simulink model "s3"  (Simulink 2.00)
settings: Solver=ode15s  StartTime=0.0  StopTime=tstop  MaxStep=1e-3  RelTol=1e-6  AbsTol=1e-6
values from neighbouring files (symbols this model uses):
  Domega = 0    [P20HP.M]
  H = J*wbm*wbm/(2*Sb)    (= 3.33396824273)    [P20HP.M]
  lambdadre = lambdadr.*(invspeed.*mask + notmask)    [M3.M]
  P = 4    [P20HP.M]
  Psidso = 0    [M1C.M]    (also in M1O.M; M3.M)
  Psipdro = 0    [M1C.M]    (also in M1O.M; M3.M)
  Psipqro = 0    [M1C.M]    (also in M1O.M; M3.M)
  Psiqso = 0    [M1C.M]    (also in M1O.M; M3.M)
  rpr = 0.0764    [P20HP.M]
  rs = 0.1062    [P20HP.M]
  speed = wbm*speed    [M3.M]
  speed_wref = [0 0.5 0.5 -0.5 -0.5 0]    [M1C.M]    (also in M1O.M = [0 1 1]; M3.M = [0 wbm/2 wbm/2 -wbm/2 -wbm/2 0])
  Tfactor = (3*P)/(4*wb)    (= 0.00795774715459)    [P20HP.M]
  time_tmech = [0 4]    [M1C.M]    (also in M1O.M = [0 0.75 0.75 1.0 1.0 1.25 1.25 1.5 1.5 2]; M3.M = [0 tstop])
  time_wref = [0 0.25 0.5 1.0 1.25 1.5]    [M1C.M]    (also in M1O.M = [0 0.5 4]; M3.M)
  tmech_tmech = [0 0]    [M1C.M]    (also in M1O.M = [0 0 -Trated -Trated -Trated/2 -Trated/2 -Trated -Trated 0 0; M3.M)
  wb = 2*pi*frated    (= 376.991118431)    [P20HP.M]
  wrbywbo = 0    [M1C.M]    (also in M1O.M; M3.M)
  xls = (we/wb)*xls    [M1C.M]    (also in M1O.M; M3.M; P20HP.M = 0.2145)
  xm = (we/wb)*xm    [M1C.M]    (also in M1O.M; M3.M; P20HP.M = 5.8339)
  xM = 1/(1/xm + 1/xls + 1/xplr)    [M1C.M]    (also in M1O.M; M3.M; P20HP.M = 0.105313916498)
  xplr = (we/wb)*xplr    [M1C.M]    (also in M1O.M; M3.M; P20HP.M = 0.2145)
  xr = xplr + xm    [M1C.M]    (also in M1O.M; M3.M)
  Zb = Vrated*Vrated/Sb    (= 3.24396782842)    [P20HP.M]
settings Model: SaveTime=off  SaveOutput=off  ConsistencyChecking=off

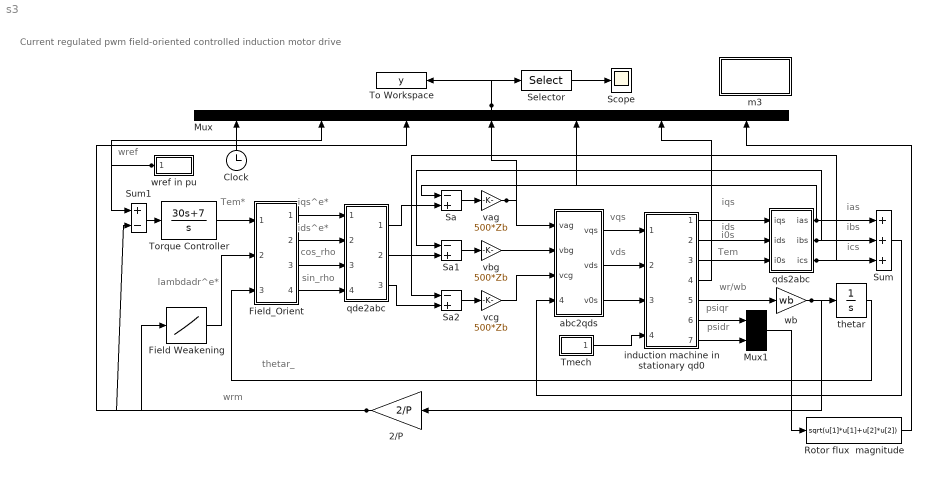
== system s3 ==
  note: Current regulated pwm
      | field-oriented controlled
      | induction motor drive
  note: Tem*
  note: cos_rho
  note: iqs^e*
  note: wref
  note: wrm
  note: thetar_
  note: ids^e*
  note: ics
  note: ibs
  note: ias
  note: vqs
  note: vds
  note: iqs
  note: ids
  note: Tem
  note: wr/wb
  note: i0s
  note: psiqr
  note: psidr
  note: lambdadr^e*
  note: sin_rho
  2/P : Gain  Orientation=left  Gain=2/P
  Clock : Clock
      settings: Orientation=up  DeleteFcn=simclock BlockIsBeingDestroyed  PostSaveFcn=simclock Save
  Field Weakening : Lookup  InputValues=speed  OutputValues=lambdadre
  Field_Orient : Subsystem
  m3 : Subsystem
      settings: OpenFcn=m3
      mask Type: Masked block of m3.m
      mask Help: Uses m3.m to initialize and plot
      mask Display: disp('Initialize\nand plot')
  Mux : Mux  Orientation=up  Inputs=7
  Mux1 : Mux  Inputs=2
  Rotor flux  magnitude : Fcn  Expr=sqrt(u[1]*u[1]+u[2]*u[2])
  Sa : Sum  Inputs=-+
  Sa1 : Sum  Inputs=-+
  Sa2 : Sum  Inputs=-+
  Scope : Scope
      settings: TickLabels=on  TimeRange=2  YMin=-200  YMax=200  SaveToWorkspace=off  SaveName=ScopeData  LimitMaxRows=off
  Selector : Selector  Elements=[3 4 5 6 7]  InputPortWidth=7
  Sum : Sum  Inputs=+++
  Sum1 : Sum  Inputs=+-
  Tmech : Subsystem  mask(Repeating table){rep_seq_t=time_tmech, rep_seq_y=tmech_tmech}
      mask prompts: rep_seq_t "Time values:"; rep_seq_y "Output values:"
      mask help: Repeating table.
      mask init:
      | period = max(rep_seq_t);
      mask Help: Repeats cycle given in table. Time values should be monotonically increasing.
      mask Display: plot([rep_seq_t,rep_seq_t+period,rep_seq_t+2*period,rep_seq_t(1)+3*period],[rep_seq_y,rep_seq_y,rep_seq_y,rep_seq_y(1)])
  To Workspace : ToWorkspace  VariableName=y  SampleTime=0
      settings: Buffer=40000
  Torque Controller : TransferFcn  Numerator=[30 7]  Denominator=[1 0]
  abc2qds : Subsystem
  induction machine in stationary qd0 : Subsystem
  qde2abc : Subsystem
  qds2abc : Subsystem
  thetar : Integrator  ExternalReset=none  InitialConditionSource=internal  InitialCondition=0  LimitOutput=off  UpperSaturationLimit=inf  LowerSaturationLimit=-inf  ShowSaturationPort=off  ShowStatePort=off  AbsoluteTolerance=auto
  vag : Gain  Gain=500*Zb
  vbg : Gain  Gain=500*Zb
  vcg : Gain  Gain=500*Zb
  wb : Gain  Gain=wb
  wref in pu : Subsystem  Orientation=left  mask(Repeating table){rep_seq_t=time_wref, rep_seq_y=speed_wref}
      mask prompts: rep_seq_t "Time values:"; rep_seq_y "Output values:"
      mask help: Repeating table.
      mask init:
      | period = max(rep_seq_t);
      mask Help: Repeats cycle given in table. Time values should be monotonically increasing.
      mask Display: plot([rep_seq_t,rep_seq_t+period,rep_seq_t+2*period,rep_seq_t(1)+3*period],[rep_seq_y,rep_seq_y,rep_seq_y,rep_seq_y(1)])
  wires:
  wref in pu/1(out_1) -> Mux/2, Sum1/1
  Tmech/1(out_1) -> induction machine in stationary qd0/4(in_Tmech)
  Mux/1 -> Selector/1, To Workspace/1
  Selector/1 -> Scope/1
  Sum1/1 -> Torque Controller/1
  Torque Controller/1 -> Field_Orient/1(Tem*)
  vag/1 -> Mux/4, abc2qds/1(vag)
  vcg/1 -> abc2qds/3(vcg)
  vbg/1 -> abc2qds/2(vbg)
  Field Weakening/1 -> Field_Orient/2(lambdadre)
  Rotor flux  magnitude/1 -> Mux/7
  induction machine in stationary qd0/4(out_Tem) -> Mux/6
  qde2abc/2(ibs*) -> Sa1/2
  Mux1/1 -> Rotor flux  magnitude/1
  induction machine in stationary qd0/7(out_psidr) -> Mux1/2
  induction machine in stationary qd0/6(out_psiqr) -> Mux1/1
  Sa2/1 -> vcg/1
  Sa/1 -> vag/1
  Sa1/1 -> vbg/1
  2/P/1 -> Mux/3, Sum1/2, Field Weakening/1
  wb/1 -> 2/P/1, thetar/1
  thetar/1 -> Field_Orient/3(thetar)
  qds2abc/3(ics) -> Sa2/1, Sum/3
  qds2abc/2(ibs) -> Sa1/1, Sum/2
  qds2abc/1(ias) -> Mux/5, Sa/1, Sum/1
  qde2abc/3(ics*) -> Sa2/2
  qde2abc/1(ias*) -> Sa/2
  Field_Orient/4(sin_rho) -> qde2abc/4(sin_rho)
  Field_Orient/3(cos_rho) -> qde2abc/3(cos_rho)
  Field_Orient/2(ids^e*) -> qde2abc/2(ids^e*)
  Field_Orient/1(iqs^e*) -> qde2abc/1(iqs^e*)
  induction machine in stationary qd0/5(out_wr/wb) -> wb/1
  induction machine in stationary qd0/3(out_i0s) -> qds2abc/3(i0s)
  induction machine in stationary qd0/2(out_ids) -> qds2abc/2(ids)
  induction machine in stationary qd0/1(out_iqs) -> qds2abc/1(iqs)
  abc2qds/2(vds) -> induction machine in stationary qd0/2(in_vds)
  Sum/1 -> abc2qds/4(ias+ibs+ics)
  Clock/1 -> Mux/1
  abc2qds/1(vqs) -> induction machine in stationary qd0/1(in_vqs)
  abc2qds/3(v0s) -> induction machine in stationary qd0/3(in_v0s)

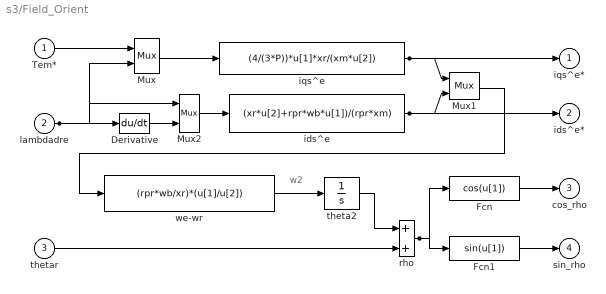
== system s3/Field_Orient ==
  note: w2
  Tem* : Inport  Port=1  PortWidth=-1  SampleTime=-1
  lambdadre : Inport  Port=2  PortWidth=-1  SampleTime=-1
  thetar : Inport  Port=3  PortWidth=-1  SampleTime=-1
  Derivative : Derivative
  Fcn : Fcn  Expr=cos(u[1])
  Fcn1 : Fcn  Expr=sin(u[1])
  Mux : Mux  Inputs=2
  Mux1 : Mux  Inputs=2
  Mux2 : Mux  Inputs=2
  ids^e : Fcn  Expr=(xr*u[2]+rpr*wb*u[1])/(rpr*xm)
  iqs^e : Fcn  Expr=(4/(3*P))*u[1]*xr/(xm*u[2])
  rho : Sum  Inputs=++
  theta2 : Integrator  ExternalReset=none  InitialConditionSource=internal  InitialCondition=0  LimitOutput=off  UpperSaturationLimit=inf  LowerSaturationLimit=-inf  ShowSaturationPort=off  ShowStatePort=off  AbsoluteTolerance=auto
  we-wr : Fcn  Expr=(rpr*wb/xr)*(u[1]/u[2])
  iqs^e* : Outport  Port=1  InitialOutput=0
  ids^e* : Outport  Port=2  InitialOutput=0
  cos_rho : Outport  Port=3  InitialOutput=0
  sin_rho : Outport  Port=4  InitialOutput=0
  wires:
  ids^e/1 -> Mux1/2, ids^e*/1
  Mux2/1 -> ids^e/1
  lambdadre/1 -> Mux2/1, Mux/2, Derivative/1
  Fcn1/1 -> sin_rho/1
  thetar/1 -> rho/2
  Fcn/1 -> cos_rho/1
  iqs^e/1 -> iqs^e*/1, Mux1/1
  Tem*/1 -> Mux/1
  Mux/1 -> iqs^e/1
  Mux1/1 -> we-wr/1
  we-wr/1 -> theta2/1
  theta2/1 -> rho/1
  rho/1 -> Fcn/1, Fcn1/1
  Derivative/1 -> Mux2/2

== system s3/m3 ==
  note: Masked block of m3.m to initialize s3.m
      | and plot results of the simulation

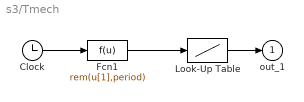
== system s3/Tmech ==
  Clock : Clock
      settings: DeleteFcn=simclock BlockIsBeingDestroyed  PostSaveFcn=simclock Save
  Fcn1 : Fcn  Expr=rem(u[1],period)
  Look-Up Table : Lookup  InputValues=rep_seq_t  OutputValues=rep_seq_y
  out_1 : Outport  Port=1  InitialOutput=0
  wires:
  Look-Up Table/1 -> out_1/1
  Clock/1 -> Fcn1/1
  Fcn1/1 -> Look-Up Table/1

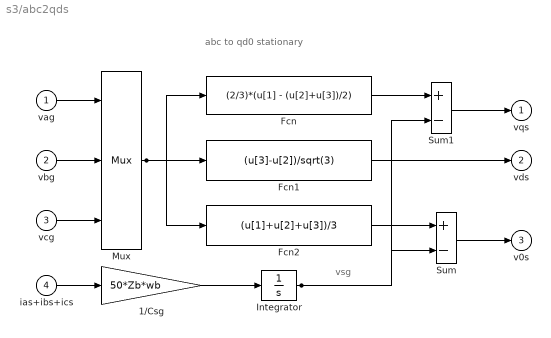
== system s3/abc2qds ==
  note: vsg
  note: abc to qd0 stationary
  vag : Inport  Port=1  PortWidth=-1  SampleTime=-1
  vbg : Inport  Port=2  PortWidth=-1  SampleTime=-1
  vcg : Inport  Port=3  PortWidth=-1  SampleTime=-1
  ias+ibs+ics : Inport  Port=4  PortWidth=-1  SampleTime=-1
  1/Csg : Gain  Gain=50*Zb*wb
  Fcn : Fcn  Expr=(2/3)*(u[1] - (u[2]+u[3])/2)
  Fcn1 : Fcn  Expr=(u[3]-u[2])/sqrt(3)
  Fcn2 : Fcn  Expr=(u[1]+u[2]+u[3])/3
  Integrator : Integrator  ExternalReset=none  InitialConditionSource=internal  InitialCondition=0  LimitOutput=off  UpperSaturationLimit=inf  LowerSaturationLimit=-inf  ShowSaturationPort=off  ShowStatePort=off  AbsoluteTolerance=auto
  Mux : Mux  Inputs=3
  Sum : Sum  Inputs=+-
  Sum1 : Sum  Inputs=+-
  vqs : Outport  Port=1  InitialOutput=0
  vds : Outport  Port=2  InitialOutput=0
  v0s : Outport  Port=3  InitialOutput=0
  wires:
  Integrator/1 -> Sum1/2, Sum/2
  Sum1/1 -> vqs/1
  Fcn/1 -> Sum1/1
  1/Csg/1 -> Integrator/1
  Fcn2/1 -> Sum/1
  Sum/1 -> v0s/1
  Fcn1/1 -> vds/1
  Mux/1 -> Fcn2/1, Fcn/1, Fcn1/1
  vcg/1 -> Mux/3
  vbg/1 -> Mux/2
  vag/1 -> Mux/1
  ias+ibs+ics/1 -> 1/Csg/1

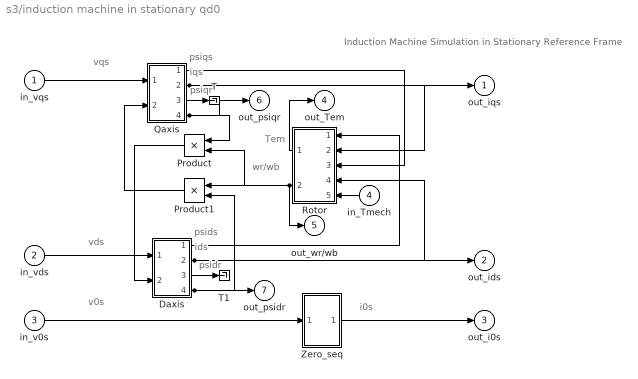
== system s3/induction machine in stationary qd0 ==
  note: Induction Machine Simulation
      |   in Stationary Reference Frame
  note: psiqs
  note: iqs
  note: psiqr
  note: psids
  note: psidr
  note: ids
  note: vqs
  note: vds
  note: wr/wb
  note: Tem
  note: i0s
  note: v0s
  in_vqs : Inport  Port=1  PortWidth=-1  SampleTime=-1
  in_vds : Inport  Port=2  PortWidth=-1  SampleTime=-1
  in_v0s : Inport  Port=3  PortWidth=-1  SampleTime=-1
  in_Tmech : Inport  Orientation=left  Port=4  PortWidth=-1  SampleTime=-1
  Daxis : Subsystem
  Product : Product  Orientation=left  Inputs=2
  Product1 : Product  Orientation=left  Inputs=2
  Qaxis : Subsystem
  Rotor : Subsystem  Orientation=left
  T : Terminator
  T1 : Terminator
  Zero_seq : Subsystem
  out_iqs : Outport  Port=1  InitialOutput=0
  out_ids : Outport  Port=2  InitialOutput=0
  out_i0s : Outport  Port=3  InitialOutput=0
  out_Tem : Outport  Port=4  InitialOutput=0
  out_wr/wb : Outport  Port=5  InitialOutput=0
  out_psiqr : Outport  Port=6  InitialOutput=0
  out_psidr : Outport  Port=7  InitialOutput=0
  wires:
  Daxis/3(out_idr') -> T1/1
  Qaxis/3(out_iqr') -> T/1
  Daxis/4(out_psidr') -> Product1/2, out_psidr/1
  Qaxis/4(out_psiqr') -> Product/1, out_psiqr/1
  Rotor/2(out_wr/wb) -> Product1/1, Product/2, out_wr/wb/1
  Daxis/1(out_psids) -> Rotor/1(in_psids)
  Product/1 -> Daxis/2(in_(wr/wb)*psiqr')
  Qaxis/2(out_iqs) -> Rotor/2(in_iqs), out_iqs/1
  Qaxis/1(out_psiqs) -> Rotor/3(in_psiqs)
  Product1/1 -> Qaxis/2(in_(wr/wb)*psidr')
  Daxis/2(out_ids) -> Rotor/4(in_ids), out_ids/1
  Rotor/1(out_Tem) -> out_Tem/1
  in_Tmech/1 -> Rotor/5(in_Tmech)
  in_vqs/1 -> Qaxis/1(in_vqs)
  in_v0s/1 -> Zero_seq/1(in_v0s)
  in_vds/1 -> Daxis/1(in_vds)
  Zero_seq/1(out_i0s) -> out_i0s/1

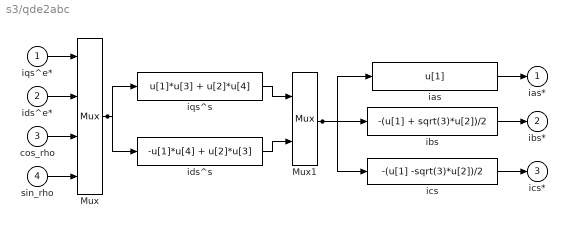
== system s3/qde2abc ==
  iqs^e* : Inport  Port=1  PortWidth=-1  SampleTime=-1
  ids^e* : Inport  Port=2  PortWidth=-1  SampleTime=-1
  cos_rho : Inport  Port=3  PortWidth=-1  SampleTime=-1
  sin_rho : Inport  Port=4  PortWidth=-1  SampleTime=-1
  Mux : Mux  Inputs=4
  Mux1 : Mux  Inputs=2
  ias : Fcn  Expr=u[1]
  ibs : Fcn  Expr=-(u[1] + sqrt(3)*u[2])/2
  ics : Fcn  Expr=-(u[1] -sqrt(3)*u[2])/2
  ids^s : Fcn  Expr=-u[1]*u[4] + u[2]*u[3]
  iqs^s : Fcn  Expr=u[1]*u[3] + u[2]*u[4]
  ias* : Outport  Port=1  InitialOutput=0
  ibs* : Outport  Port=2  InitialOutput=0
  ics* : Outport  Port=3  InitialOutput=0
  wires:
  ics/1 -> ics*/1
  sin_rho/1 -> Mux/4
  cos_rho/1 -> Mux/3
  ibs/1 -> ibs*/1
  ids^e*/1 -> Mux/2
  ias/1 -> ias*/1
  iqs^e*/1 -> Mux/1
  Mux/1 -> iqs^s/1, ids^s/1
  iqs^s/1 -> Mux1/1
  ids^s/1 -> Mux1/2
  Mux1/1 -> ias/1, ibs/1, ics/1

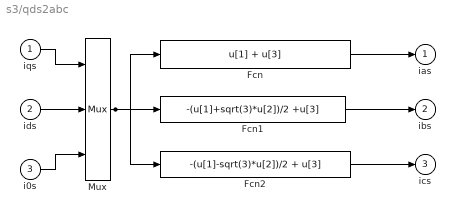
== system s3/qds2abc ==
  iqs : Inport  Port=1  PortWidth=-1  SampleTime=-1
  ids : Inport  Port=2  PortWidth=-1  SampleTime=-1
  i0s : Inport  Port=3  PortWidth=-1  SampleTime=-1
  Fcn : Fcn  Expr=u[1] + u[3]
  Fcn1 : Fcn  Expr=-(u[1]+sqrt(3)*u[2])/2 +u[3]
  Fcn2 : Fcn  Expr=-(u[1]-sqrt(3)*u[2])/2 + u[3]
  Mux : Mux  Inputs=3
  ias : Outport  Port=1  InitialOutput=0
  ibs : Outport  Port=2  InitialOutput=0
  ics : Outport  Port=3  InitialOutput=0
  wires:
  Fcn2/1 -> ics/1
  Mux/1 -> Fcn2/1, Fcn/1, Fcn1/1
  Fcn/1 -> ias/1
  Fcn1/1 -> ibs/1
  i0s/1 -> Mux/3
  iqs/1 -> Mux/1
  ids/1 -> Mux/2

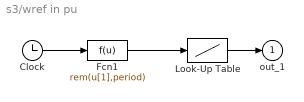
== system s3/wref in pu ==
  Clock : Clock
      settings: DeleteFcn=simclock BlockIsBeingDestroyed  PostSaveFcn=simclock Save
  Fcn1 : Fcn  Expr=rem(u[1],period)
  Look-Up Table : Lookup  InputValues=rep_seq_t  OutputValues=rep_seq_y
  out_1 : Outport  Port=1  InitialOutput=0
  wires:
  Fcn1/1 -> Look-Up Table/1
  Clock/1 -> Fcn1/1
  Look-Up Table/1 -> out_1/1

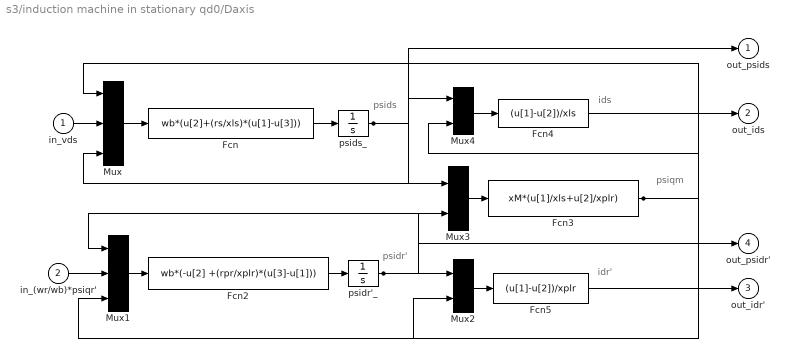
== system s3/induction machine in stationary qd0/Daxis ==
  note: ids
  note: psids
  note: psiqm
  note: idr'
  note: psidr'
  in_vds : Inport  Port=1  PortWidth=-1  SampleTime=-1
  in_(wr/wb)*psiqr' : Inport  Port=2  PortWidth=-1  SampleTime=-1
  Fcn : Fcn  Expr=wb*(u[2]+(rs/xls)*(u[1]-u[3]))
  Fcn2 : Fcn  Expr=wb*(-u[2] +(rpr/xplr)*(u[3]-u[1]))
  Fcn3 : Fcn  Expr=xM*(u[1]/xls+u[2]/xplr)
  Fcn4 : Fcn  Expr=(u[1]-u[2])/xls
  Fcn5 : Fcn  Expr=(u[1]-u[2])/xplr
  Mux : Mux  Inputs=3
  Mux1 : Mux  Inputs=3
  Mux2 : Mux  Inputs=2
  Mux3 : Mux  Inputs=2
  Mux4 : Mux  Inputs=2
  psidr'_ : Integrator  ExternalReset=none  InitialConditionSource=internal  InitialCondition=Psipdro  LimitOutput=off  UpperSaturationLimit=inf  LowerSaturationLimit=-inf  ShowSaturationPort=off  ShowStatePort=off  AbsoluteTolerance=auto
  psids_ : Integrator  ExternalReset=none  InitialConditionSource=internal  InitialCondition=Psidso  LimitOutput=off  UpperSaturationLimit=inf  LowerSaturationLimit=-inf  ShowSaturationPort=off  ShowStatePort=off  AbsoluteTolerance=auto
  out_psids : Outport  Port=1  InitialOutput=0
  out_ids : Outport  Port=2  InitialOutput=0
  out_idr' : Outport  Port=3  InitialOutput=0
  out_psidr' : Outport  Port=4  InitialOutput=0
  wires:
  Mux2/1 -> Fcn5/1
  psidr'_/1 -> Mux2/1, Mux3/2, Mux1/1, out_psidr'/1
  Mux1/1 -> Fcn2/1
  Fcn3/1 -> Mux2/2, Mux/1, Mux1/3, Mux4/2
  Mux4/1 -> Fcn4/1
  Mux3/1 -> Fcn3/1
  psids_/1 -> Mux/3, Mux4/1, Mux3/1, out_psids/1
  Fcn2/1 -> psidr'_/1
  Fcn/1 -> psids_/1
  Mux/1 -> Fcn/1
  Fcn4/1 -> out_ids/1
  in_vds/1 -> Mux/2
  in_(wr/wb)*psiqr'/1 -> Mux1/2
  Fcn5/1 -> out_idr'/1

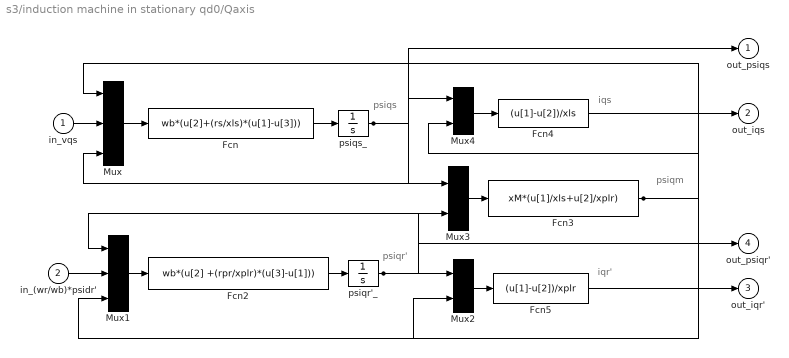
== system s3/induction machine in stationary qd0/Qaxis ==
  note: iqs
  note: psiqs
  note: psiqm
  note: iqr'
  note: psiqr'
  in_vqs : Inport  Port=1  PortWidth=-1  SampleTime=-1
  in_(wr/wb)*psidr' : Inport  Port=2  PortWidth=-1  SampleTime=-1
  Fcn : Fcn  Expr=wb*(u[2]+(rs/xls)*(u[1]-u[3]))
  Fcn2 : Fcn  Expr=wb*(u[2] +(rpr/xplr)*(u[3]-u[1]))
  Fcn3 : Fcn  Expr=xM*(u[1]/xls+u[2]/xplr)
  Fcn4 : Fcn  Expr=(u[1]-u[2])/xls
  Fcn5 : Fcn  Expr=(u[1]-u[2])/xplr
  Mux : Mux  Inputs=3
  Mux1 : Mux  Inputs=3
  Mux2 : Mux  Inputs=2
  Mux3 : Mux  Inputs=2
  Mux4 : Mux  Inputs=2
  psiqr'_ : Integrator  ExternalReset=none  InitialConditionSource=internal  InitialCondition=Psipqro  LimitOutput=off  UpperSaturationLimit=inf  LowerSaturationLimit=-inf  ShowSaturationPort=off  ShowStatePort=off  AbsoluteTolerance=auto
  psiqs_ : Integrator  ExternalReset=none  InitialConditionSource=internal  InitialCondition=Psiqso  LimitOutput=off  UpperSaturationLimit=inf  LowerSaturationLimit=-inf  ShowSaturationPort=off  ShowStatePort=off  AbsoluteTolerance=auto
  out_psiqs : Outport  Port=1  InitialOutput=0
  out_iqs : Outport  Port=2  InitialOutput=0
  out_iqr' : Outport  Port=3  InitialOutput=0
  out_psiqr' : Outport  Port=4  InitialOutput=0
  wires:
  Mux2/1 -> Fcn5/1
  psiqr'_/1 -> Mux2/1, Mux3/2, Mux1/1, out_psiqr'/1
  Mux1/1 -> Fcn2/1
  Fcn3/1 -> Mux2/2, Mux/1, Mux1/3, Mux4/2
  Mux4/1 -> Fcn4/1
  Mux3/1 -> Fcn3/1
  psiqs_/1 -> Mux/3, Mux4/1, Mux3/1, out_psiqs/1
  Fcn2/1 -> psiqr'_/1
  Fcn/1 -> psiqs_/1
  Mux/1 -> Fcn/1
  Fcn4/1 -> out_iqs/1
  in_vqs/1 -> Mux/2
  in_(wr/wb)*psidr'/1 -> Mux1/2
  Fcn5/1 -> out_iqr'/1

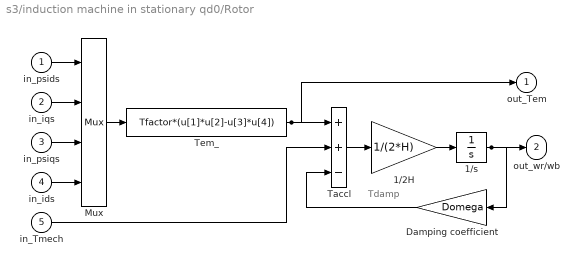
== system s3/induction machine in stationary qd0/Rotor ==
  note: Tdamp
  in_psids : Inport  Port=1  PortWidth=-1  SampleTime=-1
  in_iqs : Inport  Port=2  PortWidth=-1  SampleTime=-1
  in_psiqs : Inport  Port=3  PortWidth=-1  SampleTime=-1
  in_ids : Inport  Port=4  PortWidth=-1  SampleTime=-1
  in_Tmech : Inport  Port=5  PortWidth=-1  SampleTime=-1
  1/2H : Gain  Gain=1/(2*H)
  1/s : Integrator  ExternalReset=none  InitialConditionSource=internal  InitialCondition=wrbywbo  LimitOutput=off  UpperSaturationLimit=inf  LowerSaturationLimit=-inf  ShowSaturationPort=off  ShowStatePort=off  AbsoluteTolerance=auto
  Damping coefficient : Gain  Orientation=left  Gain=Domega
  Mux : Mux  Inputs=4
  Taccl : Sum  Inputs=++-
  Tem_ : Fcn  Expr=Tfactor*(u[1]*u[2]-u[3]*u[4])
  out_Tem : Outport  Port=1  InitialOutput=0
  out_wr/wb : Outport  Port=2  InitialOutput=0
  wires:
  1/s/1 -> out_wr/wb/1, Damping coefficient/1
  in_Tmech/1 -> Taccl/2
  Taccl/1 -> 1/2H/1
  1/2H/1 -> 1/s/1
  Tem_/1 -> Taccl/1, out_Tem/1
  Damping coefficient/1 -> Taccl/3
  Mux/1 -> Tem_/1
  in_psids/1 -> Mux/1
  in_iqs/1 -> Mux/2
  in_psiqs/1 -> Mux/3
  in_ids/1 -> Mux/4

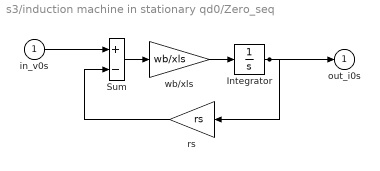
== system s3/induction machine in stationary qd0/Zero_seq ==
  in_v0s : Inport  Port=1  PortWidth=-1  SampleTime=-1
  Integrator : Integrator  ExternalReset=none  InitialConditionSource=internal  InitialCondition=0  LimitOutput=off  UpperSaturationLimit=inf  LowerSaturationLimit=-inf  ShowSaturationPort=off  ShowStatePort=off  AbsoluteTolerance=auto
  Sum : Sum  Inputs=+-
  rs : Gain  Orientation=left  Gain=rs
  wb/xls : Gain  Gain=wb/xls
  out_i0s : Outport  Port=1  InitialOutput=0
  wires:
  rs/1 -> Sum/2
  Integrator/1 -> rs/1, out_i0s/1
  Sum/1 -> wb/xls/1
  wb/xls/1 -> Integrator/1
  in_v0s/1 -> Sum/1
